simulink model "Deliverable"  (R2020a)
settings: Solver=FixedStepAuto  StartTime=0.0  StopTime=10.0  FixedStep=1e-3  RelTol=1e-3  EnableMultiTasking=on
undefined symbols (not defined in the file or in its folder): A0, A1, D0, D1, D10, D11, D12, D13, D2, D3, D4, D5, D6, D7, D8, D9, PTA0, PTA1, PTA2, PTB2, PTB23, PTB3, PTB9, PTC16, PTC17, PTC2, PTC3, PTC4, PTD0, PTD1, PTD2, PTD3
libraries: frdmk64flib x21, etargetslib x4, simulink x2
settings Model: ExtModeTrigDuration=5  Creator=shivr  LastModifiedBy=shivr
settings OptimizationCC: EnhancedBackFolding=on  PassReuseOutputArgsAs=Individual arguments  ZeroExternalMemoryAtStartup=off  ZeroInternalMemoryAtStartup=off  MaxStackSize=64  OptimizeBlockOrder=speed  DifferentSizesBufferReuse=on  OptimizationCustomize=off  EfficientTunableParamExpr=on
settings DebuggingCC: ParameterTunabilityLossMsg=error
settings HardwareCC: ProdBitPerPointer=32  ProdBitPerSizeT=32  ProdBitPerPtrDiffT=32  ProdLargestAtomicInteger=Long  ProdLargestAtomicFloat=Double  ProdWordSize=32  ProdHWDeviceType=ARM Compatible->ARM Cortex
settings SFSimCC: MATLABDynamicMemAlloc=off
settings RTWCC: SystemTargetFile=ert.tlc  HardwareBoard=NXP FRDM-K64F  TemplateMakefile=ert_default_tmf  Toolchain=GNU Tools for ARM Embedded Processors
settings CodeAppCC: ForceParamTrailComments=on  IgnoreCustomStorageClasses=off  OperatorAnnotations=on  SimulinkDataObjDesc=on  SFDataObjDesc=on  InsertBlockDesc=on

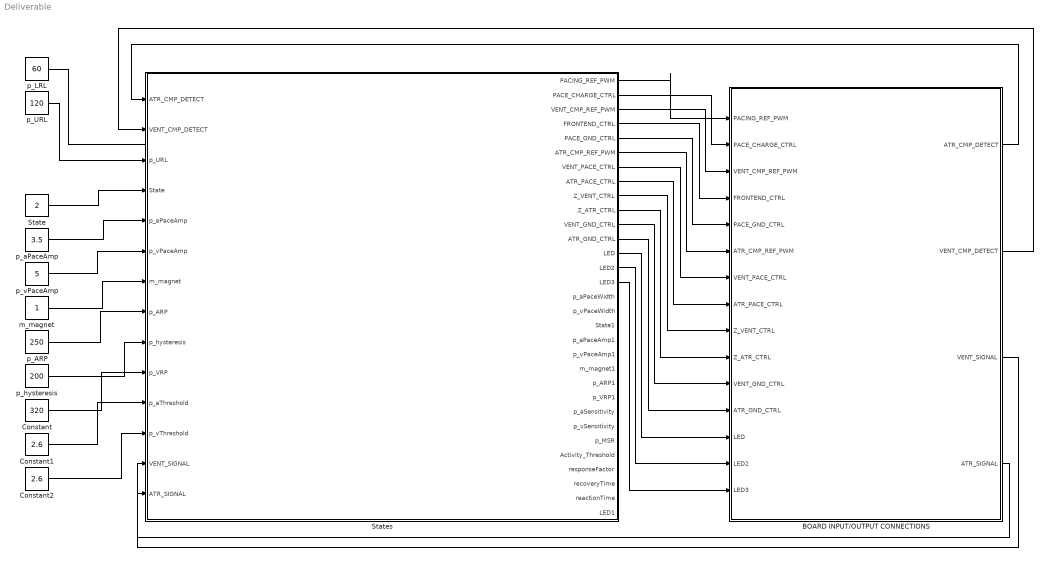
== system Deliverable ==
  BOARD INPUT/OUTPUT CONNECTIONS : Subsystem
  Constant : Constant  Value=320
  Constant1 : Constant  Value=2.6
  Constant2 : Constant  Value=2.6
  State : Constant  Value=2
  States : Subsystem
  m_magnet : Constant
  p_ARP : Constant  Value=250
  p_LRL : Constant  Value=60
  p_URL : Constant  Value=120
  p_aPaceAmp : Constant  Value=3.5
  p_hysteresis : Constant  Value=200
  p_vPaceAmp : Constant  Value=5
  wires:
  p_LRL/1 -> ?
  States/12(ATR_GND_CTRL) -> BOARD INPUT/OUTPUT CONNECTIONS/12(ATR_GND_CTRL)
  States/5(PACE_GND_CTRL) -> BOARD INPUT/OUTPUT CONNECTIONS/5(PACE_GND_CTRL)
  States/11(VENT_GND_CTRL) -> BOARD INPUT/OUTPUT CONNECTIONS/11(VENT_GND_CTRL)
  States/7(VENT_PACE_CTRL) -> BOARD INPUT/OUTPUT CONNECTIONS/7(VENT_PACE_CTRL)
  States/8(ATR_PACE_CTRL) -> BOARD INPUT/OUTPUT CONNECTIONS/8(ATR_PACE_CTRL)
  States/9(Z_VENT_CTRL) -> BOARD INPUT/OUTPUT CONNECTIONS/9(Z_VENT_CTRL)
  States/10(Z_ATR_CTRL) -> BOARD INPUT/OUTPUT CONNECTIONS/10(Z_ATR_CTRL)
  States/4(FRONTEND_CTRL) -> BOARD INPUT/OUTPUT CONNECTIONS/4(FRONTEND_CTRL)
  States/2(PACE_CHARGE_CTRL) -> BOARD INPUT/OUTPUT CONNECTIONS/2(PACE_CHARGE_CTRL)
  States/1(PACING_REF_PWM) -> BOARD INPUT/OUTPUT CONNECTIONS/1(PACING_REF_PWM)
  States/13(LED) -> BOARD INPUT/OUTPUT CONNECTIONS/13(LED)
  p_URL/1 -> States/3(p_URL)
  BOARD INPUT/OUTPUT CONNECTIONS/1(ATR_CMP_DETECT) -> States/1(ATR_CMP_DETECT)
  BOARD INPUT/OUTPUT CONNECTIONS/2(VENT_CMP_DETECT) -> States/2(VENT_CMP_DETECT)
  p_aPaceAmp/1 -> States/5(p_aPaceAmp)
  m_magnet/1 -> States/7(m_magnet)
  States/14(LED2) -> BOARD INPUT/OUTPUT CONNECTIONS/14(LED2)
  p_vPaceAmp/1 -> States/6(p_vPaceAmp)
  States/6(ATR_CMP_REF_PWM) -> BOARD INPUT/OUTPUT CONNECTIONS/6(ATR_CMP_REF_PWM)
  p_ARP/1 -> States/8(p_ARP)
  p_hysteresis/1 -> States/9(p_hysteresis)
  States/15(LED3) -> BOARD INPUT/OUTPUT CONNECTIONS/15(LED3)
  States/3(VENT_CMP_REF_PWM) -> BOARD INPUT/OUTPUT CONNECTIONS/3(VENT_CMP_REF_PWM)
  Constant/1 -> States/10(p_VRP)
  Constant1/1 -> States/11(p_aThreshold)
  Constant2/1 -> States/12(p_vThreshold)
  State/1 -> States/4(State)
  BOARD INPUT/OUTPUT CONNECTIONS/3(VENT_SIGNAL) -> States/13(VENT_SIGNAL)
  BOARD INPUT/OUTPUT CONNECTIONS/4(ATR_SIGNAL) -> States/14(ATR_SIGNAL)

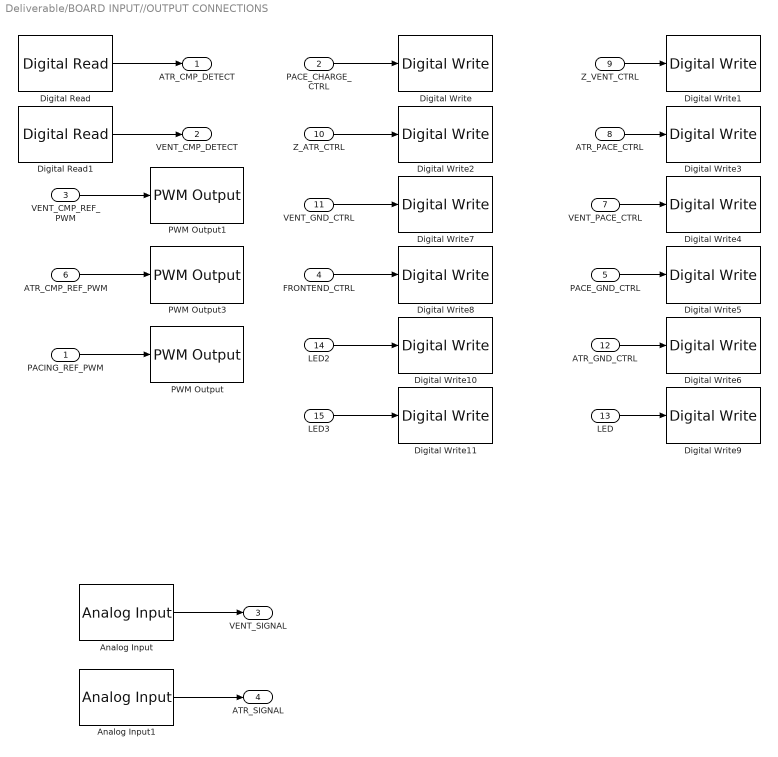
== system Deliverable/BOARD INPUT//OUTPUT CONNECTIONS ==
  PACING_REF_PWM : Inport
  PACE_CHARGE_CTRL : Inport  Port=2
  VENT_CMP_REF_PWM : Inport  Port=3
  FRONTEND_CTRL : Inport  Port=4
  PACE_GND_CTRL : Inport  Port=5
  ATR_CMP_REF_PWM : Inport  Port=6
  VENT_PACE_CTRL : Inport  Port=7
  ATR_PACE_CTRL : Inport  Port=8
  Z_VENT_CTRL : Inport  Port=9
  Z_ATR_CTRL : Inport  Port=10
  VENT_GND_CTRL : Inport  Port=11
  ATR_GND_CTRL : Inport  Port=12
  LED : Inport  Port=13
  LED2 : Inport  Port=14
  LED3 : Inport  Port=15
  Analog Input : frdmk64flib/Analog Input  Whichpin=PTB3 (A1)  SampleTime=-1
  Analog Input1 : frdmk64flib/Analog Input  Whichpin=PTB2 (A0)  SampleTime=-1
  Digital Read : frdmk64flib/Digital Read  Whichpin=PTC16 (D0)  SampleTime=-1
  Digital Read1 : frdmk64flib/Digital Read  Whichpin=PTC17 (D1)  SampleTime=-1
  Digital Write : frdmk64flib/Digital Write  Whichpin=PTB9 (D2)
  Digital Write1 : frdmk64flib/Digital Write  Whichpin=PTC3 (D7)
  Digital Write10 : frdmk64flib/Digital Write  Whichpin=BLUE_LED
  Digital Write11 : frdmk64flib/Digital Write  Whichpin=GREEN_LED
  Digital Write2 : frdmk64flib/Digital Write  Whichpin=PTB23 (D4)
  Digital Write3 : frdmk64flib/Digital Write  Whichpin=PTA0 (D8)
  Digital Write4 : frdmk64flib/Digital Write  Whichpin=PTC4 (D9)
  Digital Write5 : frdmk64flib/Digital Write  Whichpin=PTD0 (D10)
  Digital Write6 : frdmk64flib/Digital Write  Whichpin=PTD2 (D11)
  Digital Write7 : frdmk64flib/Digital Write  Whichpin=PTD3 (D12)
  Digital Write8 : frdmk64flib/Digital Write  Whichpin=PTD1 (D13)
  Digital Write9 : frdmk64flib/Digital Write  Whichpin=RED_LED
  PWM Output : frdmk64flib/PWM Output  Whichpin=PTA2 (D5)  InitialFrequency=2000  InitialDutyCycle=0
  PWM Output1 : frdmk64flib/PWM Output  Whichpin=PTA1 (D3)  InitialFrequency=2000  InitialDutyCycle=0
  PWM Output3 : frdmk64flib/PWM Output  Whichpin=PTC2 (D6)  InitialFrequency=2000  InitialDutyCycle=100
  ATR_CMP_DETECT : Outport
  VENT_CMP_DETECT : Outport  Port=2
  VENT_SIGNAL : Outport  Port=3
  ATR_SIGNAL : Outport  Port=4
  wires:
  Digital Read/1 -> ATR_CMP_DETECT/1
  Digital Read1/1 -> VENT_CMP_DETECT/1
  VENT_CMP_REF_PWM/1 -> PWM Output1/1
  PACE_CHARGE_CTRL/1 -> Digital Write/1
  Z_ATR_CTRL/1 -> Digital Write2/1
  PACING_REF_PWM/1 -> PWM Output/1
  ATR_CMP_REF_PWM/1 -> PWM Output3/1
  Z_VENT_CTRL/1 -> Digital Write1/1
  ATR_PACE_CTRL/1 -> Digital Write3/1
  VENT_PACE_CTRL/1 -> Digital Write4/1
  PACE_GND_CTRL/1 -> Digital Write5/1
  ATR_GND_CTRL/1 -> Digital Write6/1
  VENT_GND_CTRL/1 -> Digital Write7/1
  FRONTEND_CTRL/1 -> Digital Write8/1
  LED/1 -> Digital Write9/1
  LED2/1 -> Digital Write10/1
  LED3/1 -> Digital Write11/1
  Analog Input1/1 -> ATR_SIGNAL/1
  Analog Input/1 -> VENT_SIGNAL/1

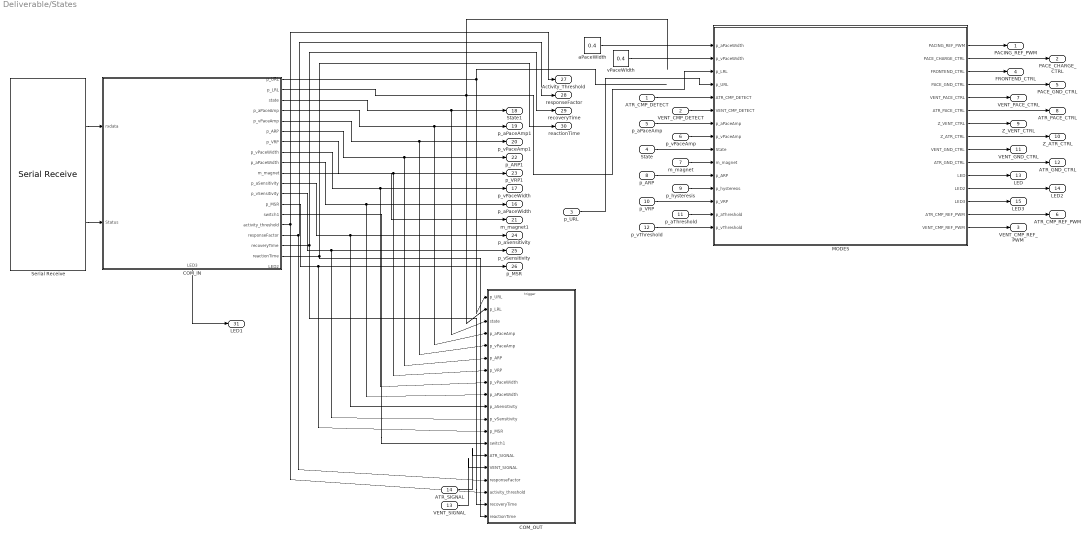
== system Deliverable/States ==
  ATR_CMP_DETECT : Inport
  VENT_CMP_DETECT : Inport  Port=2
  p_URL : Inport  Port=3
  State : Inport  Port=4
  p_aPaceAmp : Inport  Port=5
  p_vPaceAmp : Inport  Port=6
  m_magnet : Inport  Port=7
  p_ARP : Inport  Port=8
  p_hysteresis : Inport  Port=9
  p_VRP : Inport  Port=10
  p_aThreshold : Inport  Port=11
  p_vThreshold : Inport  Port=12
  VENT_SIGNAL : Inport  Port=13
  ATR_SIGNAL : Inport  Port=14
  COM_IN : Stateflow chart  TreatAsAtomicUnit=on
      settings: PortSchema="{\"entries\":[{\"content\":{\"sides\":[{\"content\":{\"connectorIds\":[\"In1\",\"In2\"]},\"type\":\"ConnectorPlacement.EquallySpacedRectSide\",\"uuid\":\"681f57b6-49ac-4d80-9ab2-cad3bca82375\"},{\"content\":{\"connectorIds\":[\"Out2\",\"Out3\",\"Out4\",\"Out5\",\"Out6\",\"Out7\",\"Out8\",\"Out9\",\"Out10\",\"Out11\",\"Out13\",\"Out12\",\"Out14\",\"Out15\",\"Out16\",\"Out17\",\"Out18\",\"Out19\",\"Out20\"],\"side\":\"RIGHT\"},\"type\":\"ConnectorPlacement.EquallySpacedRectSide\",\"uuid\":\"1cdce91e-0dc8-4b82-ba23-01e034c78730\"},{\"content\":{\"connectorIds\":[],\"side\":\"TOP\"},\"type\":\"ConnectorPlacement.EquallySpacedRectSide\",\"uuid\":\"17be7155-86f5-4b23-bee0-ec98ad7a6ec3\"},{\"content\":{\"connectorIds\":[\"Out1\"],\"side\":\"BOTTOM\"},\"type\":\"ConnectorPlacement.EquallySpacedRectSide\",\"uuid\":\"3f944ddf-95ac-4193-9b25-550dbec2da5e\"}]},\"type\":\"ConnectorPlacement.EquallySpacedConnector\",\"uuid\":\"44abe4ff-4688-435d-91fa-4b45d30c117c\"}],\"packageUris\":[\"http://schema.mathworks.com/mf0/Connector/19700101\"],\"version\":\"1.0\"}"
  COM_OUT : Subsystem
  MODES : Stateflow chart  TreatAsAtomicUnit=on
      settings: PortSchema="{\"entries\":[{\"content\":{\"sides\":[{\"content\":{\"connectorIds\":[\"In1\",\"In2\",\"In3\",\"In4\",\"In5\",\"In6\",\"In7\",\"In8\",\"In9\",\"In10\",\"In11\",\"In12\",\"In13\",\"In14\",\"In15\"]},\"type\":\"ConnectorPlacement.EquallySpacedRectSide\",\"uuid\":\"8502a3c5-6307-4e02-81ee-17e1a35cc298\"},{\"content\":{\"connectorIds\":[\"Out1\",\"Out2\",\"Out3\",\"Out4\",\"Out5\",\"Out6\",\"Out7\",\"Out8\",\"Out9\",\"Out10\",\"Out11\",\"Out14\",\"Out13\",\"Out12\",\"Out15\"],\"side\":\"RIGHT\"},\"type\":\"ConnectorPlacement.EquallySpacedRectSide\",\"uuid\":\"71555ad9-e88e-4949-94fd-af1b739ca2ca\"},{\"content\":{\"connectorIds\":[],\"side\":\"TOP\"},\"type\":\"ConnectorPlacement.EquallySpacedRectSide\",\"uuid\":\"f0239cae-2fc2-4d44-ac00-93735ab3ef8c\"},{\"content\":{\"connectorIds\":[],\"side\":\"BOTTOM\"},\"type\":\"ConnectorPlacement.EquallySpacedRectSide\",\"uuid\":\"7d1612d5-a202-47d8-98e6-e2ca77499232\"}]},\"type\":\"ConnectorPlacement.EquallySpacedConnector\",\"uuid\":\"0a066545-78b2-4ddc-84c3-90461cea3699\"}],\"packageUris\":[\"http://schema.mathworks.com/mf0/Connector/19700101\"],\"version\":\"1.0\"}"
  Serial Receive : frdmk64flib/Serial Receive  SCIModule=0  Baudrate=uint32(9600)  Parity=None  StopBits=1  HardwareFlowControl=None  ByteOrder=LittleEndian  DataType=uint8  DataLength=20  BlockingMode=off  OutputStatus=on  SampleTime=-1
  aPaceWidth : Constant  Value=0.4
  vPaceWidth : Constant  Value=0.4
  PACING_REF_PWM : Outport
  PACE_CHARGE_CTRL : Outport  Port=2
  VENT_CMP_REF_PWM : Outport  Port=3
  FRONTEND_CTRL : Outport  Port=4
  PACE_GND_CTRL : Outport  Port=5
  ATR_CMP_REF_PWM : Outport  Port=6
  VENT_PACE_CTRL : Outport  Port=7
  ATR_PACE_CTRL : Outport  Port=8
  Z_VENT_CTRL : Outport  Port=9
  Z_ATR_CTRL : Outport  Port=10
  VENT_GND_CTRL : Outport  Port=11
  ATR_GND_CTRL : Outport  Port=12
  LED : Outport  Port=13
  LED2 : Outport  Port=14
  LED3 : Outport  Port=15
  p_aPaceWidth : Outport  Port=16
  p_vPaceWidth : Outport  Port=17
  State1 : Outport  Port=18
  p_aPaceAmp1 : Outport  Port=19
  p_vPaceAmp1 : Outport  Port=20
  m_magnet1 : Outport  Port=21
  p_ARP1 : Outport  Port=22
  p_VRP1 : Outport  Port=23
  p_aSensitivity : Outport  Port=24
  p_vSensitivity : Outport  Port=25
  p_MSR : Outport  Port=26
  Activity_Threshold : Outport  Port=27
  responseFactor : Outport  Port=28
  recoveryTime : Outport  Port=29
  reactionTime : Outport  Port=30
  LED1 : Outport  Port=31
  wires:
  aPaceWidth/1 -> MODES/1(p_aPaceWidth)
  MODES/5(VENT_PACE_CTRL) -> VENT_PACE_CTRL/1
  MODES/3(FRONTEND_CTRL) -> FRONTEND_CTRL/1
  MODES/1(PACING_REF_PWM) -> PACING_REF_PWM/1
  MODES/6(ATR_PACE_CTRL) -> ATR_PACE_CTRL/1
  MODES/7(Z_VENT_CTRL) -> Z_VENT_CTRL/1
  MODES/4(PACE_GND_CTRL) -> PACE_GND_CTRL/1
  MODES/8(Z_ATR_CTRL) -> Z_ATR_CTRL/1
  MODES/2(PACE_CHARGE_CTRL) -> PACE_CHARGE_CTRL/1
  MODES/9(VENT_GND_CTRL) -> VENT_GND_CTRL/1
  MODES/10(ATR_GND_CTRL) -> ATR_GND_CTRL/1
  MODES/11(LED) -> LED/1
  COM_IN/2(p_URL) -> COM_OUT/1(p_URL)
  ATR_CMP_DETECT/1 -> MODES/5(ATR_CMP_DETECT)
  VENT_CMP_DETECT/1 -> MODES/6(VENT_CMP_DETECT)
  p_aPaceAmp/1 -> MODES/7(p_aPaceAmp)
  m_magnet/1 -> MODES/10(m_magnet)
  MODES/14(LED2) -> LED2/1
  vPaceWidth/1 -> MODES/2(p_vPaceWidth)
  p_vPaceAmp/1 -> MODES/8(p_vPaceAmp)
  MODES/12(ATR_CMP_REF_PWM) -> ATR_CMP_REF_PWM/1
  p_ARP/1 -> MODES/11(p_ARP)
  p_hysteresis/1 -> MODES/12(p_hysteresis)
  MODES/13(LED3) -> LED3/1
  p_VRP/1 -> MODES/13(p_VRP)
  MODES/15(VENT_CMP_REF_PWM) -> VENT_CMP_REF_PWM/1
  p_aThreshold/1 -> MODES/14(p_aThreshold)
  p_vThreshold/1 -> MODES/15(p_vThreshold)
  State/1 -> MODES/9(State)
  COM_IN/1(LED3) -> LED1/1
  COM_IN/15(switch1) -> COM_OUT/13(switch1)
  COM_IN/19(reactionTime) -> COM_OUT/19(reactionTime), reactionTime/1
  COM_IN/5(p_aPaceAmp) -> COM_OUT/4(p_aPaceAmp), p_aPaceAmp1/1
  COM_IN/10(p_aPaceWidth) -> p_aPaceWidth/1, COM_OUT/9(p_aPaceWidth)
  COM_IN/16(activity_threshold) -> COM_OUT/17(activity_threshold), Activity_Threshold/1
  VENT_SIGNAL/1 -> COM_OUT/15(VENT_SIGNAL)
  COM_IN/12(p_vSensitivity) -> COM_OUT/11(p_vSensitivity), p_vSensitivity/1
  COM_IN/14(p_MSR) -> COM_OUT/12(p_MSR), p_MSR/1
  COM_IN/18(recoveryTime) -> COM_OUT/18(recoveryTime), recoveryTime/1
  COM_IN/17(responseFactor) -> COM_OUT/16(responseFactor), responseFactor/1
  ATR_SIGNAL/1 -> COM_OUT/14(ATR_SIGNAL)
  COM_IN/11(m_magnet) -> m_magnet1/1
  COM_IN/4(state) -> COM_OUT/3(state), State1/1
  COM_IN/13(p_aSensitivity) -> p_aSensitivity/1, COM_OUT/10(p_aSensitivity)
  Serial Receive/1 -> COM_IN/1(rxdata)
  Serial Receive/2 -> COM_IN/2(Status)
  COM_IN/7(p_ARP) -> COM_OUT/6(p_ARP), p_ARP1/1
  COM_IN/9(p_vPaceWidth) -> COM_OUT/8(p_vPaceWidth), p_vPaceWidth/1
  COM_IN/6(p_vPaceAmp) -> COM_OUT/5(p_vPaceAmp), p_vPaceAmp1/1
  COM_IN/8(p_VRP) -> COM_OUT/7(p_VRP), p_VRP1/1
  COM_IN/3(p_LRL) -> MODES/3(p_LRL), COM_OUT/2(p_LRL)
  p_URL/1 -> MODES/4(p_URL)

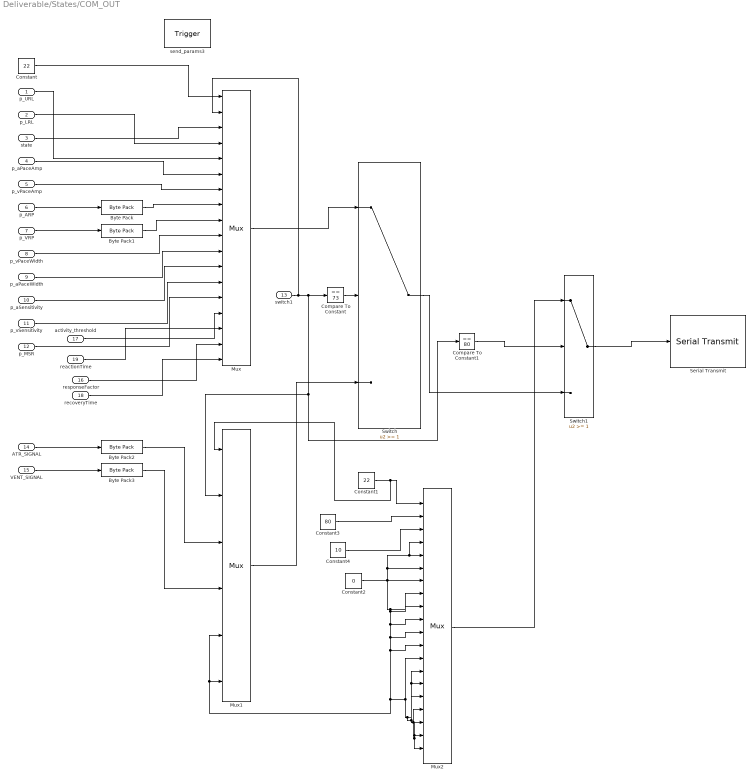
== system Deliverable/States/COM_OUT ==
  p_URL : Inport
  p_LRL : Inport  Port=2
  state : Inport  Port=3
  p_aPaceAmp : Inport  Port=4
  p_vPaceAmp : Inport  Port=5
  p_ARP : Inport  Port=6
  p_VRP : Inport  Port=7
  p_vPaceWidth : Inport  Port=8
  p_aPaceWidth : Inport  Port=9
  p_aSensitivity : Inport  Port=10
  p_vSensitivity : Inport  Port=11
  p_MSR : Inport  Port=12  OutDataTypeStr=uint8
  switch1 : Inport  Port=13
  ATR_SIGNAL : Inport  Port=14
  VENT_SIGNAL : Inport  Port=15
  responseFactor : Inport  Port=16
  activity_threshold : Inport  Port=17
  recoveryTime : Inport  Port=18
  reactionTime : Inport  Port=19
  send_params3 : TriggerPort  TriggerType=function-call  IsSimulinkFunction=on  FunctionName=send_params3  VariantControl=Variant  PortDimensions=1
  Byte Pack : etargetslib/Byte Pack  datatypes={'uint16'}  byteAlign=1
  Byte Pack1 : etargetslib/Byte Pack  datatypes={'uint16'}  byteAlign=1
  Byte Pack2 : etargetslib/Byte Pack  datatypes={'double'}  byteAlign=1
  Byte Pack3 : etargetslib/Byte Pack  datatypes={'double'}  byteAlign=1
  Compare To Constant : simulink/Logic and Bit Operations/Compare To Constant  relop===  const=73  OutDataTypeStr=boolean
  Compare To Constant1 : simulink/Logic and Bit Operations/Compare To Constant  relop===  const=80  OutDataTypeStr=boolean
  Constant : Constant  Value=22  OutDataTypeStr=uint8
  Constant1 : Constant  Value=22  OutDataTypeStr=uint8
  Constant2 : Constant  Value=0  OutDataTypeStr=uint8
  Constant3 : Constant  Value=80  OutDataTypeStr=uint8
  Constant4 : Constant  Value=10  OutDataTypeStr=uint8
  Mux : Mux  Inputs=18
  Mux1 : Mux  Inputs=6
  Mux2 : Mux  Inputs=20
  Serial Transmit : frdmk64flib/Serial Transmit  SCIModule=0  Baudrate=uint32(9600)  Parity=None  StopBits=1  HardwareFlowControl=None  ByteOrder=LittleEndian  BlockingMode=on  OutputStatus=off
  Switch : Switch  Threshold=1
  Switch1 : Switch  Threshold=1
  wires:
  p_URL/1 -> Mux/5
  p_LRL/1 -> Mux/4
  state/1 -> Mux/3
  p_aPaceAmp/1 -> Mux/6
  p_vPaceAmp/1 -> Mux/7
  p_ARP/1 -> Byte Pack/1
  Byte Pack/1 -> Mux/8
  p_VRP/1 -> Byte Pack1/1
  Byte Pack1/1 -> Mux/9
  p_vPaceWidth/1 -> Mux/10
  p_aPaceWidth/1 -> Mux/11
  Byte Pack2/1 -> Mux1/3
  ATR_SIGNAL/1 -> Byte Pack2/1
  VENT_SIGNAL/1 -> Byte Pack3/1
  Byte Pack3/1 -> Mux1/4
  p_aSensitivity/1 -> Mux/12
  p_vSensitivity/1 -> Mux/13
  p_MSR/1 -> Mux/14
  Mux/1 -> Switch/1
  Mux1/1 -> Switch/3
  switch1/1 -> Mux/2, Compare To Constant/1, Mux1/2, Compare To Constant1/1
  Compare To Constant/1 -> Switch/2
  Compare To Constant1/1 -> Switch1/2
  Constant1/1 -> Mux1/1, Mux2/1
  Constant2/1 -> Mux2/9, Mux1/5, Mux1/6, Mux2/20, Mux2/19, Mux2/18, Mux2/17, Mux2/16, Mux2/14, Mux2/15, Mux2/13, Mux2/12, Mux2/11, Mux2/10, Mux2/8, Mux2/7, Mux2/4, Mux2/5, Mux2/6
  Mux2/1 -> Switch1/1
  Constant4/1 -> Mux2/3
  Constant3/1 -> Mux2/2
  activity_threshold/1 -> Mux/15
  reactionTime/1 -> Mux/16
  responseFactor/1 -> Mux/17
  recoveryTime/1 -> Mux/18
  Switch1/1 -> Serial Transmit/1
  Switch/1 -> Switch1/3
  Constant/1 -> Mux/1

== stateflow chart Deliverable/States/COM_IN ==
  settings: executeAtInitialization=1  initializeOutput=1
  state set_param
    entry:
    switch1 = rxdata(2);
    p_LRL = rxdata(4);
    p_URL = rxdata(5);
    state = rxdata(3);
    p_aPaceAmp = rxdata(6);
    p_vPaceAmp = rxdata(7);
    p_ARP = typecast(rxdata(8:9), 'uint16');
    p_VRP = typecast(rxdata(10:11), 'uint16');
    p_aPaceWidth = rxdata(12);
    p_vPaceWidth = rxdata(13);
    p_aSensitivity = rxdata(14);
    p_vSensitivity = rxdata(15);
    p_MSR = rxdata(16);
    LED2 = false;
    LED3= false;
    activity_threshold = rxdata(17);
    reactionTime = rxdata(18);
    responseFactor = rxdata(19);
    recoveryTime = rxdata(20);
  state Nominal
    entry:
    p_LRL = 30;
    p_URL = 120;
    state = 1;
    p_aPaceAmp = 5;
    p_vPaceAmp = 5;
    p_ARP = 250;
    p_VRP = 250;
    p_aPaceWidth = 1;
    p_vPaceWidth = 1;
    m_magnet = 0;
    p_aSensitivity = 0;
    p_vSensitivity = 0;
    p_MSR = 0;
    switch1 = 0;
    activity_threshold = 0;
    reactionTime = 30;
    responseFactor = 8;
    recoveryTime = 5;
  state egram
    entry:
    switch1 = rxdata(2);
    send_params3();
  state Standby
    entry:
    %LED3 = true;
  state Check
    entry:
    switch1 = rxdata(2);
    send_params3();
    % LED2 = true;
  state echo_param
    entry:
    switch1 = rxdata(2);
    send_params3();
    %LED2 = true;
    LED3 = false;
  set_param -> Standby
  (default) -> Nominal
  (junction 9) -> set_param [order 1] : [rxdata(2) == hex2dec ('55')]
  (junction 9) -> egram [order 3] : [rxdata(2) == hex2dec ('47')]
  (junction 10) -> (junction 9) : [rxdata(1)==hex2dec('16')]
  Nominal -> Standby
  Standby -> (junction 10) : [Status == 0]
  (junction 9) -> Check [order 4] : [rxdata(2) == hex2dec('50')]
  (junction 9) -> echo_param [order 2] : [rxdata(2) == hex2dec ('49')]
  egram -> Standby
  Check -> Standby
  echo_param -> Standby
  data: LED3 output; rxdata input uint8 size=20; p_URL output uint8; p_LRL output uint8; Status input uint8; state output uint8; p_aPaceAmp output uint8; p_vPaceAmp output uint8; p_ARP output uint16; p_VRP output uint16; p_vPaceWidth output uint8; p_aPaceWidth output uint8; m_magnet output uint8; p_vSensitivity output uint8; p_aSensitivity output uint8; p_MSR output uint8; switch1 output uint8; activity_threshold output uint8; responseFactor output uint8; recoveryTime output uint8; reactionTime output uint8; LED2 output

== stateflow chart Deliverable/States/MODES ==
  state AOO
    state Prep
      entry:
      FRONTEND_CTRL=false;                              %sensing off
      %start charging C22
      ATR_PACE_CTRL = false;                    %Dont pace Atrium
      VENT_PACE_CTRL = false;         %Vent pacing off in AOO
      %convert pace amp into a duty cycle
      PACING_REF_PWM = p_aPaceAmp/5*100;
      PACE_CHARGE_CTRL = true;   %start charging capacitor
      %discharge blocking (combined state)
      PACE_GND_CTRL = true;    %connect ground to capacitor
      Z_ATR_CTRL= false;        %disable zeroing in atr and vent
      Z_VENT_CTRL=false;
      ATR_GND_CTRL = true;               %connects atrial ground
      VENT_GND_CTRL = false;  %disconnect ventricle ground
      LED = false;                                                 % turn off LED
    state Pace
      entry:
      PACE_CHARGE_CTRL = false;   %stop charging C
      ATR_PACE_CTRL = true;                   %pace atrium
      ATR_GND_CTRL = false;         %disconnect ground
      LED = true;                                   %flash the red led
    (default) -> Prep
    Prep -> Pace : [after(60000/p_LRL-p_aPaceWidth, msec)]
    Pace -> Prep : [after(p_aPaceWidth, msec)]
  state VOO
    state VOO_Prep_State
      entry:
      FRONTEND_CTRL=false;                          %sensing off
      %charging
      ATR_PACE_CTRL = false;                 %dont pace atrium
      VENT_PACE_CTRL=false;                   %dont pace vent
      %convert vPaceAmp into duty cycle
      PACING_REF_PWM = p_vPaceAmp/5*100;
      PACE_CHARGE_CTRL=true;                %start charging
      %discharging
      PACE_GND_CTRL=true;             %connect C to ground
      Z_ATR_CTRL = false; %disable zeroing for atr and vent
      Z_VENT_CTRL=false;
      ATR_GND_CTRL = false;    %disconnect atrium ground
      VENT_GND_CTRL=true;      %connect ventricle ground
      LED2 = false;                                 % turn off blue LED
    state VOO_Pace_State
      entry:
      PACE_CHARGE_CTRL=false; %stop charging C
      VENT_GND_CTRL=false; %unground ventricle
      VENT_PACE_CTRL=true; %pace ventricle
      LED2 = true; %turn on blue LED
    (default) -> VOO_Prep_State
    VOO_Prep_State -> VOO_Pace_State : [after(60000.0/p_LRL - p_vPaceWidth,msec)]
    VOO_Pace_State -> VOO_Prep_State : [after(p_vPaceWidth,msec)]
  state state_selector
  state AAI
    state AAI_CHARGING_DISCHARGING
      entry:
      FRONTEND_CTRL = true; %enable sensing
      %charge capacitor exactly like AOO
      ATR_PACE_CTRL = false;
      PACE_CHARGE_CTRL = true;
      PACE_GND_CTRL = true;
      VENT_PACE_CTRL = false;
      PACING_REF_PWM = p_aPaceAmp/5*100;
      %discharge
      ATR_GND_CTRL = true;
      VENT_PACE_CTRL = false;
      VENT_GND_CTRL = false;
      Z_ATR_CTRL = false;
      Z_VENT_CTRL = false;
      LED3 = false;
      %set the reference comparison PWM
      ATR_CMP_REF_PWM = p_aThreshold/5*100;
    state AAI_PACING
      entry:
      %turn off sensing
      FRONTEND_CTRL = false;
      %Pace like aoo
      PACE_CHARGE_CTRL = false;
      ATR_PACE_CTRL = true;
      ATR_GND_CTRL = false;
      LED3 = true;
    state AAI_REFRACTORY
      entry:
      %enter refractory if natural atrium pulse
      % is detected and wait for p_ARP
      LED2 = ~LED2;
    (default) -> AAI_CHARGING_DISCHARGING
    AAI_CHARGING_DISCHARGING -> AAI_PACING [order 1] : [ATR_CMP_DETECT==false&&after((60000/p_LRL-p_aPaceWidth), msec)]
    AAI_PACING -> AAI_CHARGING_DISCHARGING : [after(p_aPaceWidth, msec)]
    AAI_REFRACTORY -> AAI_CHARGING_DISCHARGING : [after(p_ARP, msec)]
    AAI_CHARGING_DISCHARGING -> AAI_REFRACTORY [order 2] : [ATR_CMP_DETECT == true]
  state VVI
    state VVI_SENSING
      entry:
      FRONTEND_CTRL = true; %enable sensing
      %charge and discharge exactly like VOO
      ATR_PACE_CTRL = false;
      PACE_CHARGE_CTRL = true;
      PACE_GND_CTRL = true;
      VENT_PACE_CTRL = false;
      PACING_REF_PWM = p_vPaceAmp/5*100;
      %discharge
      ATR_GND_CTRL =false;
      VENT_GND_CTRL = true;
      Z_ATR_CTRL = false;
      Z_VENT_CTRL = false;
      LED3 = false;
      %Set the comparison reference PWM
      VENT_CMP_REF_PWM = p_vThreshold/5*100;
    state VVI_PACING
      entry:
      %turn off sensing
      FRONTEND_CTRL = false;
      %pace like VOO
      PACE_CHARGE_CTRL = false;
      PACE_GND_CTRL = true;
      VENT_PACE_CTRL = true;
      VENT_GND_CTRL = false;
      LED3 = true;
    state VVI_REFRACTORY
      entry:
      %if ventricle pulse is detected:
      %wait p_VRP
      LED2 = ~LED2;
    (default) -> VVI_SENSING
    VVI_SENSING -> VVI_PACING [order 1] : [VENT_CMP_DETECT==false&&after((60000/p_LRL-p_vPaceWidth), msec)]
    VVI_PACING -> VVI_SENSING : [after(p_vPaceWidth, msec)]
    VVI_REFRACTORY -> VVI_SENSING : [after(p_VRP, msec)]
    VVI_SENSING -> VVI_REFRACTORY [order 2] : [VENT_CMP_DETECT == true]
  state_selector -> AOO [order 1] : [State == 1&&m_magnet==0]
  state_selector -> VOO [order 2] : [m_magnet == 1 || State == 2]
  (default) -> state_selector
  state_selector -> AAI [order 3] : [State == 3&&m_magnet==0]
  state_selector -> VVI [order 4] : [State == 4&&m_magnet==0]
  data: PACING_REF_PWM output; PACE_CHARGE_CTRL output; FRONTEND_CTRL output; PACE_GND_CTRL output; VENT_PACE_CTRL output; ATR_PACE_CTRL output; Z_VENT_CTRL output; Z_ATR_CTRL output; VENT_GND_CTRL output; ATR_GND_CTRL output; LED output; ATR_CMP_REF_PWM output; LED3 output; p_aPaceWidth input; p_vPaceWidth input; p_LRL input; p_URL input; ATR_CMP_DETECT input; VENT_CMP_DETECT input; p_aPaceAmp input; p_vPaceAmp input; State input; m_magnet input; LED2 output; p_ARP input; p_hysteresis input; p_VRP input; VENT_CMP_REF_PWM output; p_aThreshold input; p_vThreshold input
